simulink model "Asservissement_Moteur"  (R2015a)
settings: Solver=ode45  StartTime=0.0  StopTime=2  MaxStep=0.0001  RelTol=1e-3
settings Model: Creator=Xavier  LastModifiedBy=Xavier

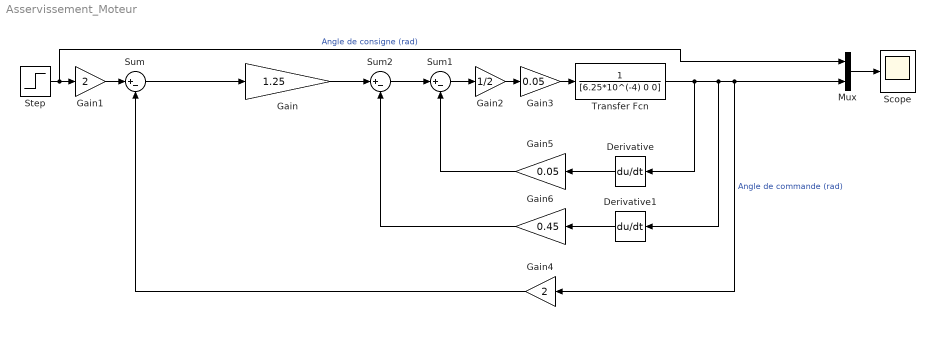
== system Asservissement_Moteur ==
  Derivative : Derivative
  Derivative1 : Derivative
  Gain : Gain  Gain=1.25
  Gain1 : Gain  Gain=2
  Gain2 : Gain  Gain=1/2
  Gain3 : Gain  Gain=0.05
  Gain4 : Gain  Gain=2
  Gain5 : Gain  Gain=0.05
  Gain6 : Gain  Gain=0.45
  Mux : Mux  Inputs=2
  Scope : Scope
      settings: ShowLegends=on  TimeRange=2  YMin=1.241095890410959  YMax=2.041095890410959
  Step : Step  Time=0  After=2  SampleTime=0
  Sum : Sum  Inputs=|+-
  Sum1 : Sum  Inputs=|+-
  Sum2 : Sum  Inputs=|+-
  Transfer Fcn : TransferFcn  Denominator=[6.25*10^(-4) 0 0]
  wires:
  Sum/1 -> Gain/1
  Gain1/1 -> Sum/1
  Sum1/1 -> Gain2/1
  Gain2/1 -> Gain3/1
  Gain3/1 -> Transfer Fcn/1
  Transfer Fcn/1 -> Derivative/1, Derivative1/1, Mux/2, Gain4/1  "Angle de commande (rad)"
  Gain5/1 -> Sum1/2
  Gain4/1 -> Sum/2
  Derivative/1 -> Gain5/1
  Sum2/1 -> Sum1/1
  Gain/1 -> Sum2/1
  Gain6/1 -> Sum2/2
  Derivative1/1 -> Gain6/1
  Step/1 -> Mux/1, Gain1/1  "Angle de consigne (rad)"
  Mux/1 -> Scope/1
